simulink model "fault_analysis"  (R2014b)
settings: Solver=ode23tb  StartTime=0.0  StopTime=1  RelTol=1e-3
undefined symbols (not defined in the file): D1, Delta
libraries: powerlib x7, powerlib_meascontrol x3, simulink_extras x3
settings Model: Creator=Amr Saleh  LastModifiedBy=Amr Saleh

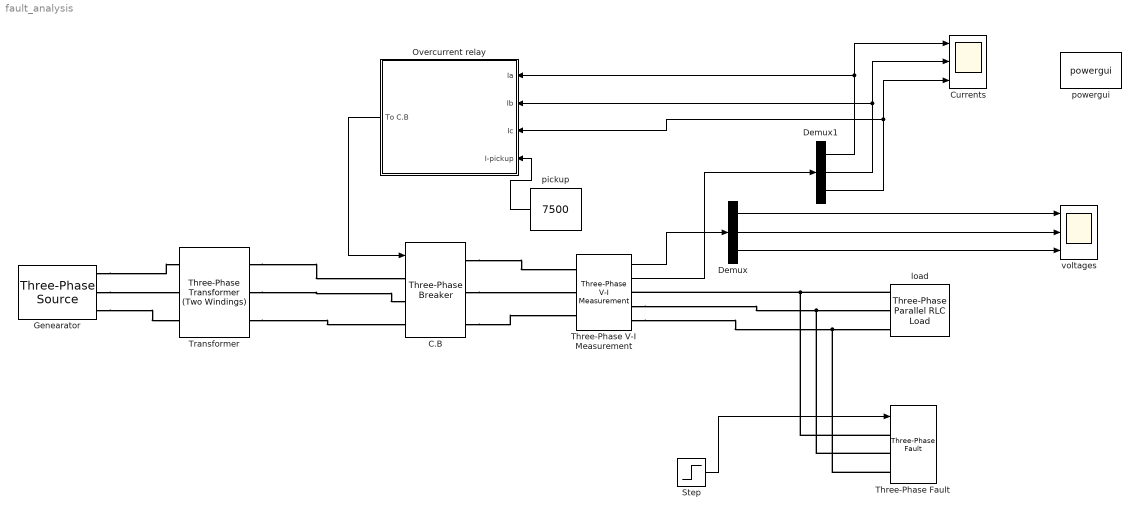
== system fault_analysis ==
  C.B : powerlib/Elements/Three-Phase Breaker  InitialState=closed  SwitchA=on  SwitchB=on  SwitchC=on  SwitchTimes="[1/60  5/60]"  External=on  BreakerResistance=0.01  SnubberResistance=1e6  SnubberCapacitance=inf  Measurements=None
  Currents : Scope  NumInputPorts=3
      settings: YMin=-5~-5~-5  YMax=5~5~5
  Demux : Demux  Outputs=3
  Demux1 : Demux  Outputs=3
  Genearator : powerlib/Electrical Sources/Three-Phase Source  Voltage=11e3  PhaseAngle=0  Frequency=50  InternalConnection=Yg  SpecifyImpedance=on  Resistance=0.8929  Inductance=16.58e-3  ShortCircuitLevel=20e6  BaseVoltage=11e3  XRratio=7  BusType=swing  Pref=0  Qref=0  Qmin=-inf  Qmax=inf
  Overcurrent relay : Subsystem
  Step : Step  Time=0.1  SampleTime=0
  Three-Phase V-I Measurement : powerlib/Measurements/Three-Phase V-I Measurement  VoltageMeasurement=phase-to-ground  SetLabelV=off  LabelV=Vabc  Vpu=off  VpuLL=off  CurrentMeasurement=yes  SetLabelI=off  LabelI=Iabc  Ipu=off  Pbase=100e6  Vbase=500e3  OutputType=Complex  PhasorSimulation=off  PSBequivalent=0
  Three-Phase Fault : powerlib/Elements/Three-Phase Fault  InitialStates=0  FaultA=on  FaultB=on  FaultC=on  GroundFault=on  SwitchTimes="[1/60  5/60]"  External=on  SwitchStatus=NaN  FaultResistance=0.001  GroundResistance=0.01  SnubberResistance=1e6  SnubberCapacitance=inf  Measurements=None
  Transformer : powerlib/Elements/Three-Phase Transformer (Two Windings)  Winding1Connection=Delta (D1)  UNITS=pu  NominalPower=[ 10e6 , 50 ]  Winding1=[ 11e3 , 0.002 , 0.08 ]  Winding2Connection=Yg  Winding2=[ 0.4e3 , 0.002 , 0.08 ]  SetSaturation=off  Rm=500  Lm=500  Saturation=[ 0,0 ; 0.0024,1.2 ; 1.0,1.52 ]  Hysteresis=off  DataFile='hysteresis'  SetInitialFlux=off  InitialFluxes=[ 0.8 , -0.8 , 0.7 ]  Measurements=None  MoreParameters=off  BreakLoop=off  DataType=off  TransfoNumber=1
  load : powerlib/Elements/Three-Phase Parallel RLC Load  LConnTagsString=A|B|C  Configuration=Y (grounded)  NominalVoltage=0.4e3  NominalFrequency=50  ActivePower=5e6  InductivePower=20e3  CapacitivePower=0  Measurements=None  LoadType=constant Z
  pickup : Constant  Value=7500  OutDataTypeStr=boolean
  powergui : powerlib/powergui  Priority=1  SimulationMode=Continuous  SolverType=Tustin/Backward Euler (TBE)  SampleTime=50e-6  frequency=60  SPID=off  DisableSnubberDevices=off  DisableRonSwitches=off  DisableVfSwitches=off  SwTol=0  DisplayEquations=off  Interpol=off  methode=off  Ts=100  frequencyindice=50  Pbase=100e6  ErrMax=1e-4  Iterations=50  UnitsV=kV  UnitsW=MW  FunctionMessages=off  echomessages=off  HookPort=off  EnableUseOfTLC=off  x0status=blocks  RestoreLinks=warning  ResistiveCurrentMeasurement=off  Frange=[0:2:500]  Ylog=off  Xlog=on  ShowGrid=off  save=off  variable=ZData  structure=0  ZoomFFT=off  StartTime=0.0  cycles=1  DisplayStyle=1  fundamental=60  FreqAxis=off  MaxFrequency=1000  frequencyindicesteady=1  RmsSteady=1  display=off
  voltages : Scope  NumInputPorts=3
      settings: YMin=-5~-5~-5  YMax=5~5~5
  wires:
  Three-Phase V-I Measurement/1 -> Demux/1
  Demux/1 -> voltages/1
  Demux/2 -> voltages/2
  Demux/3 -> voltages/3
  Demux1/1 -> Currents/1, Overcurrent relay/1(Ia)
  Demux1/2 -> Currents/2, Overcurrent relay/2(Ib)
  Demux1/3 -> Overcurrent relay/3(Ic), Currents/3
  Three-Phase V-I Measurement/2 -> Demux1/1
  Step/1 -> Three-Phase Fault/1
  pickup/1 -> Overcurrent relay/4(I-pickup)
  Overcurrent relay/1(To C.B) -> C.B/1
  connections:
  Genearator/RConn1 -- Transformer/LConn1
  Genearator/RConn2 -- Transformer/LConn2
  Genearator/RConn3 -- Transformer/LConn3
  load/LConn1 -- Three-Phase V-I Measurement/RConn1 -- Three-Phase Fault/LConn1
  Three-Phase V-I Measurement/RConn2 -- Three-Phase Fault/LConn2 -- load/LConn2
  Three-Phase V-I Measurement/RConn3 -- Three-Phase Fault/LConn3 -- load/LConn3
  Transformer/RConn1 -- C.B/LConn1
  Transformer/RConn2 -- C.B/LConn2
  Transformer/RConn3 -- C.B/LConn3
  C.B/RConn1 -- Three-Phase V-I Measurement/LConn1
  C.B/RConn2 -- Three-Phase V-I Measurement/LConn2
  C.B/RConn3 -- Three-Phase V-I Measurement/LConn3

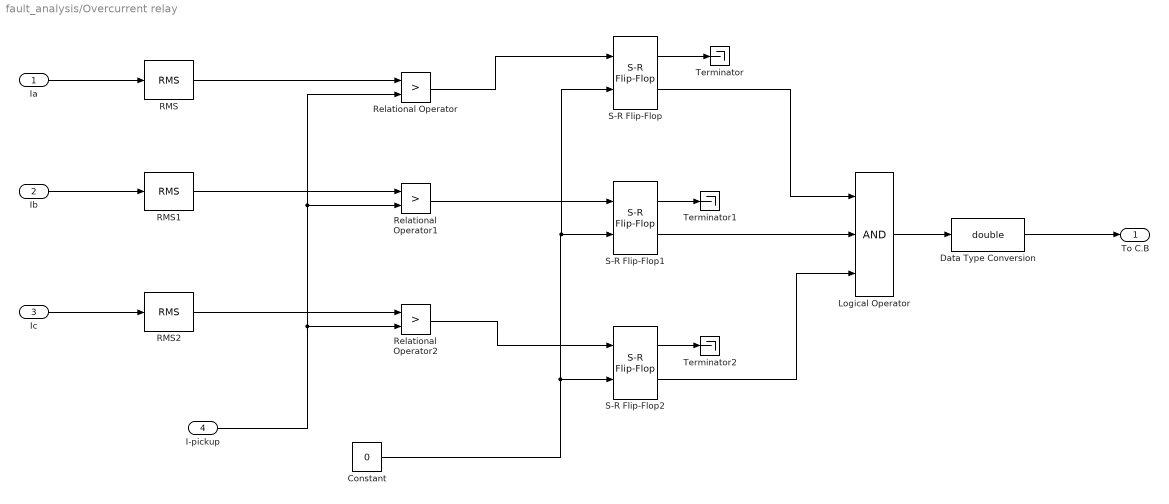
== system fault_analysis/Overcurrent relay ==
  Ia : Inport
  Ib : Inport  Port=2
  Ic : Inport  Port=3
  I-pickup : Inport  Port=4
  Constant : Constant  Value=0  OutDataTypeStr=boolean
  Data Type Conversion : DataTypeConversion  OutDataTypeStr=double
  Logical Operator : Logic  Inputs=3  AllPortsSameDT=off  OutDataTypeStr=boolean
  RMS : powerlib_meascontrol/Measurements/RMS  TrueRMS=on  Freq=50  RMSInit=0  Ts=0.5
  RMS1 : powerlib_meascontrol/Measurements/RMS  TrueRMS=on  Freq=50  RMSInit=0  Ts=0.5
  RMS2 : powerlib_meascontrol/Measurements/RMS  TrueRMS=on  Freq=50  RMSInit=0  Ts=0.5
  Relational Operator : RelationalOperator  Operator=>  OutDataTypeStr=boolean
  Relational Operator1 : RelationalOperator  Operator=>  OutDataTypeStr=boolean
  Relational Operator2 : RelationalOperator  Operator=>  OutDataTypeStr=boolean
  S-R Flip-Flop : simulink_extras/Flip Flops/S-R Flip-Flop  initial_condition=0
  S-R Flip-Flop1 : simulink_extras/Flip Flops/S-R Flip-Flop  initial_condition=0
  S-R Flip-Flop2 : simulink_extras/Flip Flops/S-R Flip-Flop  initial_condition=0
  Terminator : Terminator
  Terminator1 : Terminator
  Terminator2 : Terminator
  To C.B : Outport
  wires:
  Ia/1 -> RMS/1
  Ib/1 -> RMS1/1
  Ic/1 -> RMS2/1
  RMS/1 -> Relational Operator/1
  RMS1/1 -> Relational Operator1/1
  RMS2/1 -> Relational Operator2/1
  I-pickup/1 -> Relational Operator2/2, Relational Operator1/2, Relational Operator/2
  Constant/1 -> S-R Flip-Flop/2, S-R Flip-Flop1/2, S-R Flip-Flop2/2
  Relational Operator/1 -> S-R Flip-Flop/1
  Relational Operator1/1 -> S-R Flip-Flop1/1
  Relational Operator2/1 -> S-R Flip-Flop2/1
  S-R Flip-Flop/1 -> Terminator/1
  S-R Flip-Flop1/1 -> Terminator1/1
  S-R Flip-Flop2/1 -> Terminator2/1
  S-R Flip-Flop/2 -> Logical Operator/1
  S-R Flip-Flop1/2 -> Logical Operator/2
  S-R Flip-Flop2/2 -> Logical Operator/3
  Logical Operator/1 -> Data Type Conversion/1
  Data Type Conversion/1 -> To C.B/1
